simulink subsystem "DRV8830_Driver"  (R2022b)
settings: Solver=VariableStepAuto  StartTime=0.0  StopTime=10.0  RelTol=1e-3
model mask{driver_model=1}
  mask prompts: driver_model "Driver Parameters struct:"
settings Model: Creator=gotta  LastModifiedBy=gotta

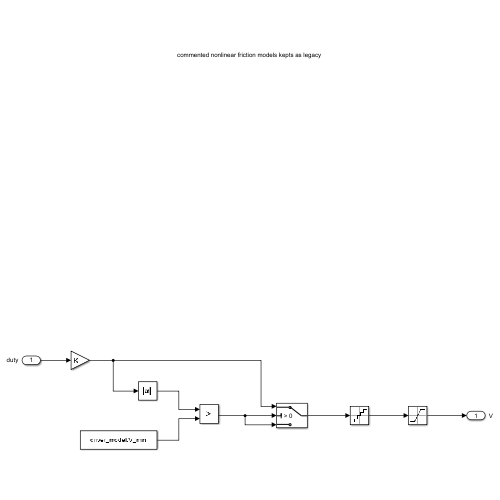
[thumbnail: Simulink's stored preview of the top-level diagram]
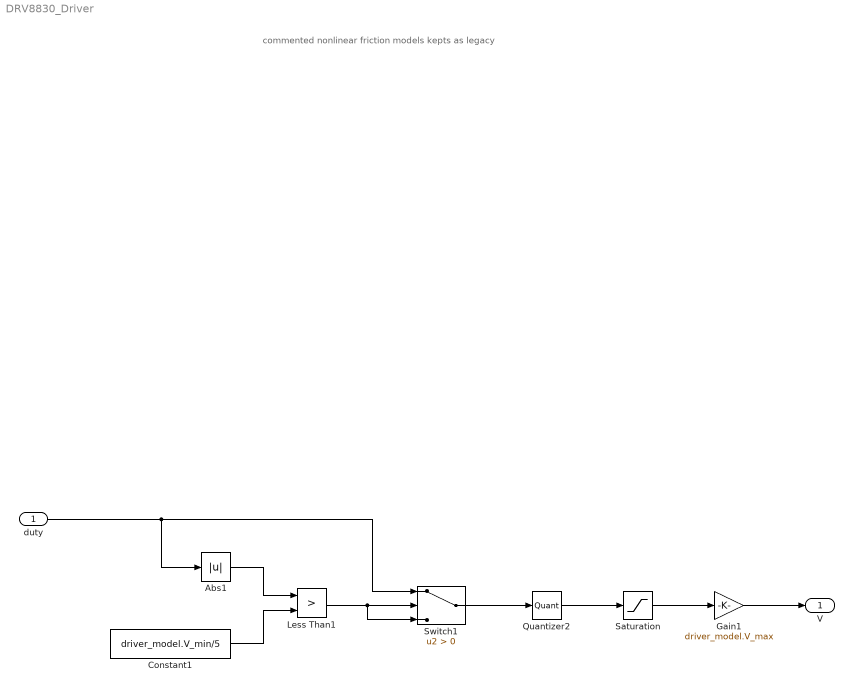
== system DRV8830_Driver ==
  note: commented nonlinear friction models kepts as legacy
  duty : Inport
  Abs1 : Abs  SaturateOnIntegerOverflow=off
  Constant1 : Constant  Value=driver_model.V_min/5
  Gain1 : Gain  Gain=driver_model.V_max
  Less Than1 : RelationalOperator  Operator=>  OutDataTypeStr=boolean  RndMeth=Simplest  InputSameDT=off
  Quantizer2 : Quantizer  QuantizationInterval=driver_model.V_step/5
  Saturation : Saturate  UpperLimit=driver_model.V_max  LowerLimit=-driver_model.V_max
  Switch1 : Switch  Criteria=u2 > Threshold  SaturateOnIntegerOverflow=off  InputSameDT=off
  V : Outport
  wires:
  Quantizer2/1 -> Saturation/1
  duty/1 -> Abs1/1, Switch1/1
  Abs1/1 -> Less Than1/1
  Constant1/1 -> Less Than1/2
  Less Than1/1 -> Switch1/3, Switch1/2
  Switch1/1 -> Quantizer2/1
  Saturation/1 -> Gain1/1
  Gain1/1 -> V/1
